simulink model "interpolation_nD_TestGen22"  (R2017b)
settings: Solver=FixedStepDiscrete  StartTime=0.0  StopTime=10.0  RelTol=1e-3
settings Model: Creator=ktrinh  LastModifiedBy=ktrinh
settings DebuggingCC: ParameterOverflowMsg=none

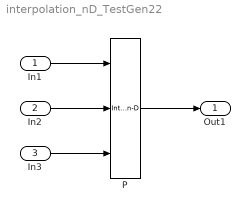
== system interpolation_nD_TestGen22 ==
  In1 : Inport  OutMax=2
  In2 : Inport  Port=2  OutMin=0  OutMax=5
  In3 : Inport  Port=3  PortDimensions=[2 5]
  P : Interpolation_n-D  TableSource=Input port  InterpMethod=Flat  NumSelectionDims=2  OutDataTypeStr=double  InternalRulePriority=Speed  RndMeth=Convergent
      settings: InputPortMap=u0,u1,p2
  Out1 : Outport
  wires:
  In1/1 -> P/1
  In2/1 -> P/2
  In3/1 -> P/3
  P/1 -> Out1/1
